simulink model "sampleModel120"  (R2021b)
settings: Solver=VariableStepAuto  StartTime=0.0  StopTime=10.0  RelTol=1e-3
undefined symbols (not defined in the file or in its folder): DiscIntNeverNeededParam, Newton, Raphson
libraries: simulink x6
settings Model: Creator=user  LastModifiedBy=user

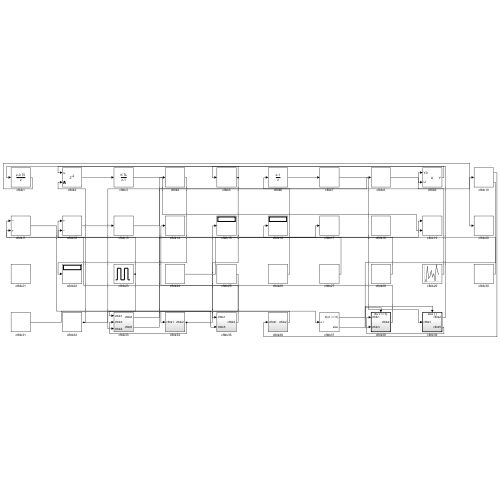
[thumbnail: Simulink's stored preview of the top-level diagram]
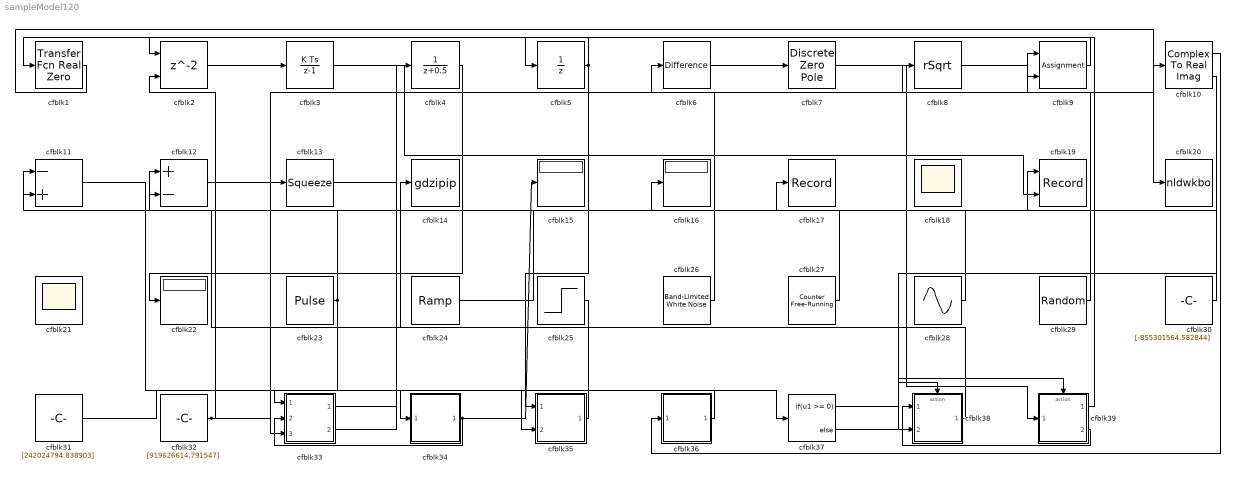
== system sampleModel120 ==
  cfblk1 : simulink/Discrete/Transfer Fcn Real Zero  ZeroZ=0.75  ICPrevInput=0.0  DoSatur=off
      settings: SourceProductBaseCode=SL
  cfblk10 : ComplexToRealImag
  cfblk11 : Sum  Inputs=-+
  cfblk12 : Sum  Inputs=+-
  cfblk13 : Squeeze
  cfblk14 : ToWorkspace  VariableName=gdzipip  SaveFormat=Timeseries  SampleTime=-1
  cfblk15 : Display
  cfblk16 : Display
  cfblk17 : Record  FileSettingsInternal="{\"entries\":[{\"content\":{\"excelSettings\":{\"content\":{},\"type\":\"Streamout.ExcelSettings\"}},\"type\":\"Streamout.FileSettingStorage\",\"uuid\":\"e0210236-c923-4f10-9e11-b856d1107aa3\"}],\"packageUris\":[\"http://schema.mathworks.com/mf0/streamout_blocks/R2020a\"],\"version\":\"1.0\"}"  SignalsInternal="{\"entries\":[{\"content\":{\"signals\":[{\"content\":{\"blockPath\":[\"sampleModel120/cfblk17\"],\"channel\":[],\"dimensions\":[1],\"domain\":\"sampleModel120/cfblk17\",\"lineColor\":\"#7e2f8e\",\"plots\":[1],\"port\":1,\"sid\":[\"\"],\"signalID\":4200,\"signalName\":\"cfblk33:2\"},\"type\":\"RecordBlkView.Signal\",\"uuid\":\"89cdf700-71f4-44c4-b849-b03ae17e177f\"}]},\"type\":\"RecordBlkView.InputSignals\",\"uuid\":\"d4e2e50f-ae13-4356-993b-0258d389af8d\"}],\"packageUris\":[\"http://schema.mathworks.com/mf0/streamout_blocks/R2020a\"],\"version\":\"1.0\"}"  VisualizationBindings="{\"sparklinesplugin\":{\"info\":[{\"bindingParametersList\":[],\"subplotID\":1}]}}"
  cfblk18 : Scope
      settings: Floating=on
  cfblk19 : Record  FileSettingsInternal="{\"entries\":[{\"content\":{\"excelSettings\":{\"content\":{},\"type\":\"Streamout.ExcelSettings\"}},\"type\":\"Streamout.FileSettingStorage\",\"uuid\":\"8366a3cd-7951-4da1-9c24-9775e92245a2\"}],\"packageUris\":[\"http://schema.mathworks.com/mf0/streamout_blocks/R2020a\"],\"version\":\"1.0\"}"  Layout=[1 1]  SignalsInternal="{\"entries\":[{\"content\":{\"signals\":[{\"content\":{\"blockPath\":[\"sampleModel120/cfblk19\"],\"channel\":[],\"dimensions\":[1],\"domain\":\"sampleModel120/cfblk19\",\"lineColor\":\"#a2142f\",\"plots\":[1],\"port\":1,\"sid\":[\"\"],\"signalID\":4204,\"signalName\":\"cfblk24\"},\"type\":\"RecordBlkView.Signal\",\"uuid\":\"4cfc79fe-18ae-4409-b2c0-2dcb3a73f501\"},{\"content\":{\"blockPath\":[\"sampleModel120/cfblk19\"],\"channel\":[],\"dimensions\":[1],\"domain\":\"sampleModel120/cfblk19\",\"lineColor\":\"#139fff\",\"plots\":[1],\"port\":2,\"sid\":[\"\"],\"signalID\":4208,\"signalName\":\"cfblk3\"},\"type\":\"RecordBlkView.Signal\",\"uuid\":\"e1144ead-9151-4cbf-b5a5-9f5ff2a6b2b2\"}]},\"type\":\"RecordBlkView.InputSignals\",\"uuid\":\"31d6f318-5164-4d5f-8776-cf26e05151e7\"}],\"packageUris\":[\"http://schema.mathworks.com/mf0/streamout_blocks/R2020a\"],\"version\":\"1.0\"}"  VisualizationBindings="{\"xyplotplugin\":{\"info\":[{\"series\":[{\"bindingParametersList\":[{\"parameter\":\"X-Axis\",\"signalID\":4204,\"signalName\":\"cfblk24\"},{\"parameter\":\"Y-Axis\",\"signalID\":4208,\"signalName\":\"cfblk3\"}],\"seriesID\":44654}],\"subplotID\":1}]}}"  CompatibilityTag=XY
  cfblk2 : Delay  ShowEnablePort=on  SampleTime=1
      settings: InputPortMap=u0,e6
  cfblk20 : ToWorkspace  VariableName=nldwkbo  SaveFormat=Timeseries  SampleTime=-1
  cfblk21 : Scope
      settings: Floating=on
  cfblk22 : Display
  cfblk23 : DiscretePulseGenerator  PulseType=Time based  Amplitude=[-795414490.972023]  Period=[15601255.876719]  PulseWidth=5  PhaseDelay=[5.000000]
  cfblk24 : simulink/Sources/Ramp  slope=[5669.634117]  start=[37.625232]  InitialOutput=[807253.537562]
  cfblk25 : Step  Time=[11.000000]  Before=[-205313429.833590]  After=[-717190819.367420]  SampleTime=0
  cfblk26 : simulink/Sources/Band-Limited White Noise  Cov=[2291830487.830296]  Ts=0.1  seed=[3676955398.000000]
  cfblk27 : simulink/Sources/Counter Free-Running  NumBits=[15.000000]  tsamp=-1
  cfblk28 : Sin  Amplitude=[156276289.097491]  Bias=[62004617.987088]  SampleTime=0
  cfblk29 : UniformRandomNumber  Minimum=[-6667408591.222454]  Maximum=[2305310778.897584]  Seed=[44039106.000000]  SampleTime=0.1
  cfblk3 : DiscreteIntegrator  ICPrevOutput=DiscIntNeverNeededParam  ICPrevScaledInput=DiscIntNeverNeededParam
  cfblk30 : Constant  Value=[-855301564.582844]  SampleTime=1
  cfblk31 : Constant  Value=[242024794.838903]  SampleTime=1
  cfblk32 : Constant  Value=[919626614.791547]  SampleTime=1
  cfblk33 : Subsystem
  cfblk34 : Subsystem
  cfblk35 : Subsystem
  cfblk36 : Subsystem
  cfblk37 : If  IfExpression=u1 >= 0  SampleTime=1
  cfblk38 : Subsystem  TreatAsAtomicUnit=on
  cfblk39 : Subsystem  TreatAsAtomicUnit=on
  cfblk4 : DiscreteTransferFcn  SampleTime=1
  cfblk5 : UnitDelay  HasFrameUpgradeWarning=on
  cfblk6 : simulink/Discrete/Difference  ICPrevInput=0.0  OutMin=[]  OutMax=[]  OutDataTypeStr=Inherit: Inherit via back propagation  OutDataType=fixdt(1, 16)  OutScaling=2^-10  DoSatur=off
  cfblk7 : DiscreteZeroPole  Poles=[0 0.5]  Gain=1
  cfblk8 : Sqrt  Operator=rSqrt  AlgorithmType=Newton-Raphson  SaturateOnIntegerOverflow=on
  cfblk9 : Assignment  DiagnosticForDimensions=Warning  IndexOptions=Index vector (dialog)  Indices=1  OutputSizes=1
  wires:
  cfblk23/1 -> cfblk11/1, cfblk33/3(cfblk4)
  cfblk29/1 -> cfblk9/1
  cfblk24/1 -> cfblk19/1
  cfblk12/1 -> cfblk13/1
  cfblk38/1(cfblk2) -> cfblk14/1
  cfblk7/1 -> cfblk39/1(cfblk1)
  cfblk36/1(cfblk2) -> cfblk33/1(cfblk1)
  cfblk39/1(cfblk2) -> cfblk5/1
  cfblk25/1 -> cfblk34/1(cfblk1)
  cfblk3/1 -> cfblk19/2
  cfblk33/1(cfblk2) -> cfblk4/1
  cfblk34/1(cfblk2) -> cfblk15/1, cfblk33/2(cfblk3)
  cfblk2/1 -> cfblk3/1
  cfblk6/1 -> cfblk7/1
  cfblk33/2(cfblk5) -> cfblk17/1
  cfblk9/1 -> cfblk1/1
  cfblk27/1 -> cfblk16/1
  cfblk39/2(cfblk5) -> cfblk38/1(cfblk1)
  cfblk8/1 -> cfblk9/2
  cfblk28/1 -> cfblk11/2
  cfblk13/1 -> cfblk8/1
  cfblk1/1 -> cfblk20/1
  cfblk30/1 -> cfblk12/1
  cfblk5/1 -> cfblk35/1(cfblk1), cfblk2/1
  cfblk10/1 -> cfblk36/1(cfblk1)
  cfblk4/1 -> cfblk22/1
  cfblk35/1(cfblk2) -> cfblk12/2
  cfblk26/1 -> cfblk6/1
  cfblk11/1 -> cfblk35/2(cfblk5)
  cfblk32/1 -> cfblk10/1, cfblk2/2
  cfblk31/1 -> cfblk37/1
  cfblk10/2 -> cfblk38/2(cfblk3)
  cfblk37/1 -> cfblk38/Action
  cfblk37/2 -> cfblk39/Action

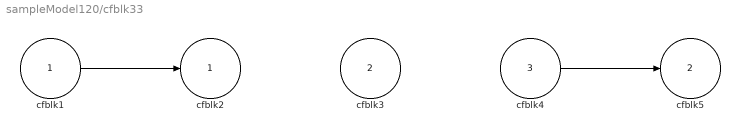
== system sampleModel120/cfblk33 ==
  cfblk1 : Inport
  cfblk3 : Inport  Port=2
  cfblk4 : Inport  Port=3
  cfblk2 : Outport
  cfblk5 : Outport  Port=2
  wires:
  cfblk1/1 -> cfblk2/1
  cfblk4/1 -> cfblk5/1

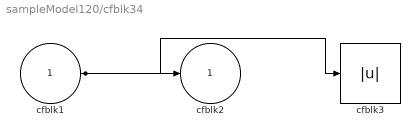
== system sampleModel120/cfblk34 ==
  cfblk1 : Inport
  cfblk3 : Abs
  cfblk2 : Outport
  wires:
  cfblk1/1 -> cfblk2/1, cfblk3/1

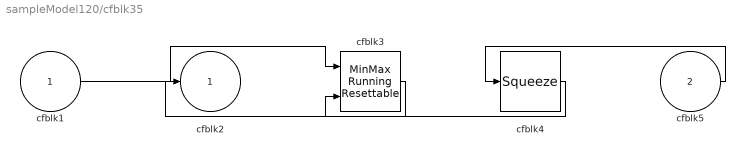
== system sampleModel120/cfblk35 ==
  cfblk1 : Inport
  cfblk5 : Inport  Port=2
  cfblk3 : simulink/Math Operations/MinMax Running Resettable  Function=min  vinit=0.0
  cfblk4 : Squeeze
  cfblk2 : Outport
  wires:
  cfblk1/1 -> cfblk3/1
  cfblk5/1 -> cfblk4/1
  cfblk3/1 -> cfblk2/1
  cfblk4/1 -> cfblk3/2

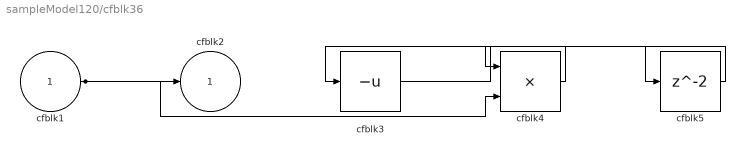
== system sampleModel120/cfblk36 ==
  cfblk1 : Inport
  cfblk3 : UnaryMinus
  cfblk4 : Product
  cfblk5 : Delay  SampleTime=1
  cfblk2 : Outport
  wires:
  cfblk1/1 -> cfblk2/1, cfblk4/2
  cfblk4/1 -> cfblk3/1
  cfblk3/1 -> cfblk5/1
  cfblk5/1 -> cfblk4/1

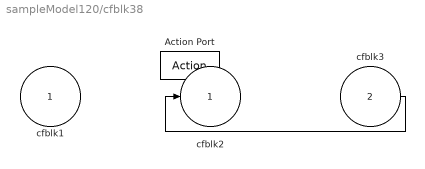
== system sampleModel120/cfblk38 ==
  cfblk1 : Inport
  cfblk3 : Inport  Port=2
  Action Port : ActionPort  ActionPortLabel=if(u1 >= 0)
  cfblk2 : Outport
  wires:
  cfblk3/1 -> cfblk2/1

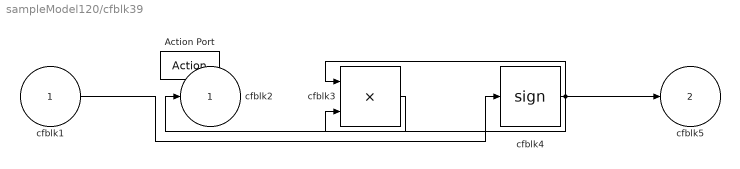
== system sampleModel120/cfblk39 ==
  cfblk1 : Inport
  Action Port : ActionPort  ActionPortLabel=else
  cfblk3 : Product  Inputs=**
  cfblk4 : Signum
  cfblk2 : Outport
  cfblk5 : Outport  Port=2
  wires:
  cfblk4/1 -> cfblk3/1, cfblk5/1, cfblk3/2
  cfblk3/1 -> cfblk2/1
  cfblk1/1 -> cfblk4/1
